simulink model "Sl_H_Infinity"  (Simulink 8.5)
settings: Solver=ode45  StartTime=0.0  StopTime=10  RelTol=1e-3
values from neighbouring files (symbols this model uses):
  Wu1 = [numu/denu]    [Sc_H_Infinity.m]
  Wu2 = [numu/denu]    [Sc_H_Infinity.m]
  Wy = [num1/den1]    [Sc_H_Infinity.m]
libraries: cstblocks x4
settings Model: Creator=jordan  LastModifiedBy=Vladislav  CovSFcnEnable=off
settings DebuggingCC: SolverPrmCheckMsg=warning  FcnCallInpInsideContextMsg=UseLocalSettings

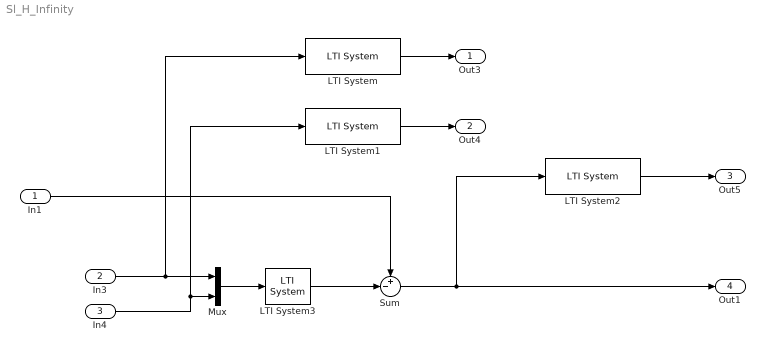
== system Sl_H_Infinity ==
  In1 : Inport
  In3 : Inport  Port=2
  In4 : Inport  Port=3
  LTI System : cstblocks/LTI System  sys=1/Wu1  IC=[]
  LTI System1 : cstblocks/LTI System  sys=1/Wu2  IC=[]
  LTI System2 : cstblocks/LTI System  sys=1/Wy  IC=[]
  LTI System3 : cstblocks/LTI System  sys=G  IC=[]
  Mux : Mux  Inputs=2
  Sum : Sum  Inputs=+-|
  Out3 : Outport
  Out4 : Outport  Port=2
  Out5 : Outport  Port=3
  Out1 : Outport  Port=4
  wires:
  In3/1 -> Mux/1, LTI System/1
  LTI System/1 -> Out3/1
  LTI System1/1 -> Out4/1
  LTI System2/1 -> Out5/1
  LTI System3/1 -> Sum/2
  Mux/1 -> LTI System3/1
  In1/1 -> Sum/1
  Sum/1 -> Out1/1, LTI System2/1
  In4/1 -> Mux/2, LTI System1/1
